simulink model "Copy_of_modelo_completo_sin_joystick"  (R2021a)
settings: Solver=FixedStepAuto  StartTime=0.0  StopTime=inf  FixedStep=0.001  MaxStep=1e-4  RelTol=1e-3
undefined symbols (not defined in the file): bah, bat, bcx, bcy, beqhd, beqt, bw, C_HEIGHT, cols_centers, cols_height, cont_mass, ddxmax, ddxmin, ddymax, ddymin, g, Kcy, Ksah, Ksat, Ksiah, Ksiat, Kw, lh0, Meqh, Meqt, mt, Rd, rt, rth, Rw, sigbuilder_block, sp_mass, VH_MAX, VT_MAX, w_mt_h, w_mt_i, xmax, xt0, ymax, yt0
libraries: simulink x1
(part 1 of 2)
settings Model: Creator=Mariano  LastModifiedBy=Mariano
settings SolverCC: ODENIntegrationMethod=ode2

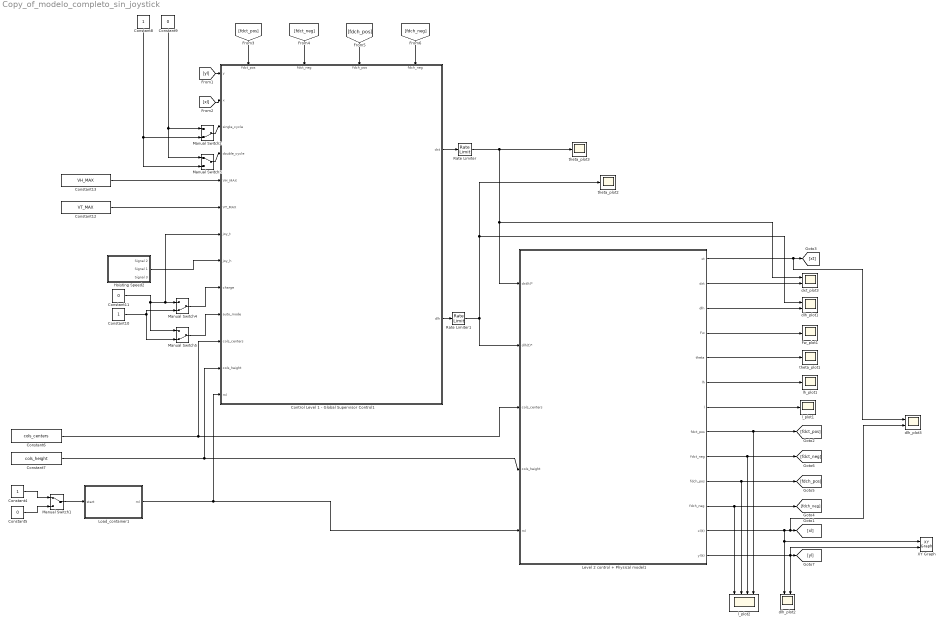
== system Copy_of_modelo_completo_sin_joystick ==
  Constant10 : Constant
  Constant11 : Constant  Value=0
  Constant12 : Constant  Value=VT_MAX
  Constant13 : Constant  Value=VH_MAX
  Constant4 : Constant
  Constant5 : Constant  Value=0
  Constant6 : Constant  Value=cols_centers
  Constant7 : Constant  Value=cols_height
  Constant8 : Constant
  Constant9 : Constant  Value=0
  Control Level 1 - Global Supervisor Control1 : Stateflow chart  TreatAsAtomicUnit=on
      settings: PortSchema="{\"entries\":[{\"content\":{\"sides\":[{\"content\":{\"connectorIds\":[\"In5\",\"In9\",\"In10\",\"In11\",\"In12\",\"In13\",\"In6\",\"In7\",\"In14\",\"In8\",\"In15\",\"In16\",\"In17\"]},\"type\":\"ConnectorPlacement.EquallySpacedRectSide\",\"uuid\":\"6e151bdd-c3d8-41a7-9f18-e2357f64189a\"},{\"content\":{\"connectorIds\":[\"Out1\",\"Out2\"],\"side\":\"RIGHT\"},\"type\":\"ConnectorPlacement.EquallySpacedRectSide\",\"uuid\":\"a3c41cfb-ae11-4b18-951d-06971f73a30a\"},{\"content\":{\"connectorIds\":[\"In1\",\"In2\",\"In3\",\"In4\"],\"side\":\"TOP\"},\"type\":\"ConnectorPlacement.EquallySpacedRectSide\",\"uuid\":\"cee4e257-0e1b-4274-aa91-a6c4290c0560\"},{\"content\":{\"connectorIds\":[],\"side\":\"BOTTOM\"},\"type\":\"ConnectorPlacement.EquallySpacedRectSide\",\"uuid\":\"f9084d8a-5b88-4444-9be3-56009c74d696\"}]},\"type\":\"ConnectorPlacement.EquallySpacedConnector\",\"uuid\":\"a9a1dd87-5328-46c3-9f4f-ca95d008ff72\"}],\"packageUris\":[\"http://schema.mathworks.com/mf0/Connector/R2020b\"],\"version\":\"1.0\"}"
  Fw_plot1 : Scope
  Hoisting Speed2 : Subsystem  Tag=STV Subsys  LoadFcn=sigbuilder_block('load',[0 30 1024.5 488.25 ]);  StartFcn=sigbuilder_block('start');  StopFcn=sigbuilder_block('stop');  ClipboardFcn=sigbuilder_block('clipboard');  mask(Sigbuilder block){tuvar=[0:10]}
      mask help: Simulink:masks:SigbuilderBlock_MD
      mask init:
      | if ~strcmp(get_param(bdroot(gcbh),'SimulationStatus'),'stopped') tuvar = sigbuilder_block('maskInit'); end
      settings: CopyFcn=sigbuilder_block('copy');  DeleteFcn=sigbuilder_block('delete');  ModelCloseFcn=sigbuilder_block('modelClose');  PreSaveFcn=sigbuilder_block('preSave');  PauseFcn=sigbuilder_block('pause');  ContinueFcn=sigbuilder_block('continue');  NameChangeFcn=sigbuilder_block('namechange');  OpenFcn=sigbuilder_block('open',[6 30 1012.5 447.75 ]);  CloseFcn=sigbuilder_block('close');
      mask Display: plot(0, 0, 100, 100,[2, 2, 32, 32, 2], [68, 8, 8, 68, 68],[32, 2], [38, 38], [32, 19, 2],[53, 60, 44], [32, 17, 17, 2],[16, 16, 31, 31]);txt = getActiveGroup(gcbh);text(2, 100, txt,'verticalAlignment', 'top');
  Level 2 control + Physical model1 : Subsystem
  Load_container1 : Subsystem
  Manual Switch1 : ManualSwitch
  Manual Switch2 : ManualSwitch  CurrentSetting=0
  Manual Switch3 : ManualSwitch
  Manual Switch4 : ManualSwitch  CurrentSetting=0
  Manual Switch5 : ManualSwitch  CurrentSetting=0
  Rate Limiter : RateLimiter  RisingSlewLimit=ddxmax  FallingSlewLimit=ddxmin  SampleTimeMode=inherited
  Rate Limiter1 : RateLimiter  RisingSlewLimit=ddymax  FallingSlewLimit=ddymin  SampleTimeMode=inherited
  XY Graph : simulink/Sinks/XY Graph  xmin=-20  xmax=60  ymin=-20  ymax=50  st=-1
  dlh_plot1 : Scope  NumInputPorts=2
  dlh_plot2 : Scope  NumInputPorts=2
  dlh_plot3 : Scope  NumInputPorts=2
  dxt_plot3 : Scope  NumInputPorts=2
  l_plot1 : Scope
  l_plot2 : Scope  NumInputPorts=4
  lh_plot1 : Scope
  theta_plot1 : Scope
  theta_plot2 : Scope
  theta_plot3 : Scope
  wires:
  [yl] -> Control Level 1 - Global Supervisor Control1/5(y)
  Manual Switch4/1 -> Control Level 1 - Global Supervisor Control1/14(charge)
  Constant11/1 -> Manual Switch5/1, Control Level 1 - Global Supervisor Control1/6(joy_t), Manual Switch4/1
  Constant9/1 -> Manual Switch3/1, Manual Switch2/1
  Manual Switch3/1 -> Control Level 1 - Global Supervisor Control1/11(double_cycle)
  Constant8/1 -> Manual Switch3/2, Manual Switch2/2
  Constant7/1 -> Level 2 control + Physical model1/4(cols_height), Control Level 1 - Global Supervisor Control1/16(cols_height)
  Constant10/1 -> Manual Switch4/2, Manual Switch5/2
  Manual Switch2/1 -> Control Level 1 - Global Supervisor Control1/10(single_cycle)
  Level 2 control + Physical model1/5(theta) -> theta_plot1/1
  Manual Switch5/1 -> Control Level 1 - Global Supervisor Control1/8(auto_mode)
  Constant5/1 -> Manual Switch1/2
  Constant13/1 -> Control Level 1 - Global Supervisor Control1/12(VH_MAX)
  Level 2 control + Physical model1/7(l) -> l_plot1/1
  Level 2 control + Physical model1/2(dxt) -> dxt_plot3/2
  Level 2 control + Physical model1/1(xt) -> dlh_plot3/1, [xt]
  Level 2 control + Physical model1/4(Fw) -> Fw_plot1/1
  Load_container1/1(ml) -> Control Level 1 - Global Supervisor Control1/17(ml), Level 2 control + Physical model1/5(ml)
  Constant12/1 -> Control Level 1 - Global Supervisor Control1/13(VT_MAX)
  Constant4/1 -> Manual Switch1/1
  Manual Switch1/1 -> Load_container1/1(start)
  [xl] -> Control Level 1 - Global Supervisor Control1/9(x)
  Level 2 control + Physical model1/3(dlh) -> dlh_plot1/2
  Level 2 control + Physical model1/6(lh) -> lh_plot1/1
  Constant6/1 -> Level 2 control + Physical model1/3(cols_centers), Control Level 1 - Global Supervisor Control1/15(cols_centers)
  Control Level 1 - Global Supervisor Control1/2(dlh) -> Rate Limiter1/1
  Control Level 1 - Global Supervisor Control1/1(dxt) -> Rate Limiter/1
  Level 2 control + Physical model1/8(fdct_pos) -> l_plot2/4, [fdct_pos]
  Level 2 control + Physical model1/9(fdct_neg) -> l_plot2/3, [fdct_neg]
  Level 2 control + Physical model1/10(fdch_pos) -> l_plot2/2, [fdch_pos]
  Level 2 control + Physical model1/11(fdch_neg) -> l_plot2/1, [fdch_neg]
  [fdct_pos] -> Control Level 1 - Global Supervisor Control1/1(fdct_pos)
  [fdct_neg] -> Control Level 1 - Global Supervisor Control1/2(fdct_neg)
  [fdch_pos] -> Control Level 1 - Global Supervisor Control1/3(fdch_pos)
  [fdch_neg] -> Control Level 1 - Global Supervisor Control1/4(fdch_neg)
  Level 2 control + Physical model1/13(yl(t)) -> XY Graph/2, dlh_plot2/2, [yl]
  Level 2 control + Physical model1/12(xl(t)) -> dlh_plot3/2, [xl], XY Graph/1, dlh_plot2/1
  Rate Limiter/1 -> theta_plot3/1, dxt_plot3/1, Level 2 control + Physical model1/1(dxt(t)*)
  Rate Limiter1/1 -> Level 2 control + Physical model1/2(dlh(t)*), theta_plot2/1, dlh_plot1/1
  Hoisting Speed2/2(Signal 1) -> Control Level 1 - Global Supervisor Control1/7(joy_h)

== system Copy_of_modelo_completo_sin_joystick/Hoisting Speed2 ==
  Demux : Demux  Tag=STV Demux  Outputs=3
      settings: DisplayOption=none
  FromWs : FromWorkspace  Tag=STV FromWs  VariableName=tuvar
      SigBuilderData=|
      | common.afterFinalStr = 'Extrapolate'
      | common.sampleTime = 0
      | dataSet.timeRange = [0 105]
      | dataSet.name = 'Group 1'
      | sbobj.Groups.Name = 'Group 1'
      | sbobj.Groups.Signals(1).Name = 'Signal 2'
      | sbobj.Groups.Signals(1).XData = [0 5 8 52 55 105]
      | sbobj.Groups.Signals(1).YData = [0 0 -1 -1 0 0]
      | sbobj.Groups.Signals(2).Name = 'Signal 1'
      | sbobj.Groups.Signals(2).XData = [0 2 4 20 22 34 36 48 50 105]
      | sbobj.Groups.Signals(2).YData = [0 0 -1 -1 0 0 1 1 0 0]
      | sbobj.Groups.Signals(3).Name = 'Signal 3'
      | sbobj.Groups.Signals(3).XData = [0 8 10 30.1 32 105]
      | sbobj.Groups.Signals(3).YData = [0 0 1 1 0 0]
      | sbobj.Groups.TimeRange = [0 105]
  Signal 2 : Outport  Tag=STV Outport
  Signal 1 : Outport  Tag=STV Outport  Port=2
  Signal 3 : Outport  Tag=STV Outport  Port=3
  wires:
  FromWs/1 -> Demux/1
  Demux/1 -> Signal 2/1
  Demux/2 -> Signal 1/1
  Demux/3 -> Signal 3/1

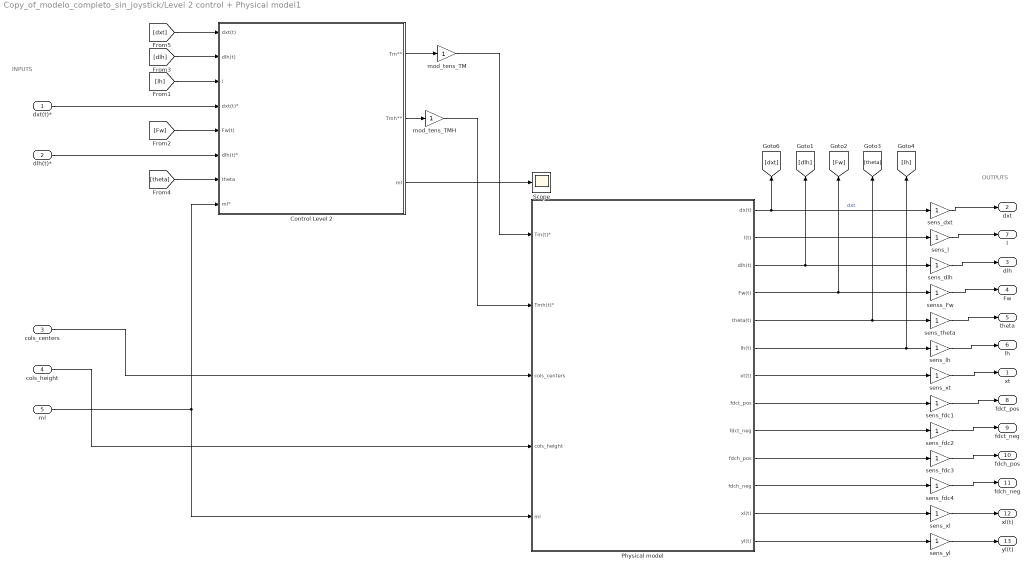
== system Copy_of_modelo_completo_sin_joystick/Level 2 control + Physical model1 ==
  note: OUTPUTS
  note: INPUTS
  dxt(t)* : Inport
  dlh(t)* : Inport  Port=2
  cols_centers : Inport  Port=3
  cols_height : Inport  Port=4
  ml : Inport  Port=5
  Control Level 2 : Subsystem
  Physical model : Subsystem
  Scope : Scope
  mod_tens_TM : Gain
  mod_tens_TMH : Gain
  sens_dlh : Gain
  sens_dxt : Gain
  sens_fdc{1..4} (4 alike) : Gain
  sens_l : Gain
  sens_lh : Gain
  sens_theta : Gain
  sens_xl : Gain
  sens_xt : Gain
  sens_yl : Gain
  senss_Fw : Gain
  xt : Outport
  dxt : Outport  Port=2
  dlh : Outport  Port=3
  Fw : Outport  Port=4
  theta : Outport  Port=5
  lh : Outport  Port=6
  l : Outport  Port=7
  fdct_pos : Outport  Port=8
  fdct_neg : Outport  Port=9
  fdch_pos : Outport  Port=10
  fdch_neg : Outport  Port=11
  xl(t) : Outport  Port=12
  yl(t) : Outport  Port=13
  wires:
  Physical model/4(Fw(t)) -> senss_Fw/1, [Fw]
  Physical model/3(dlh(t)) -> sens_dlh/1, [dlh]
  dxt(t)*/1 -> Control Level 2/4(dxt(t)*)
  senss_Fw/1 -> Fw/1
  Control Level 2/3(ml) -> Scope/1
  sens_xt/1 -> xt/1
  dlh(t)*/1 -> Control Level 2/6(dlh(t)*)
  Physical model/5(theta(t)) -> sens_theta/1, [theta]
  mod_tens_TMH/1 -> Physical model/2(Tmh(t)*)
  Physical model/1(dx(t)) -> sens_dxt/1, [dxt]  "dxt"
  ml/1 -> Physical model/5(ml), Control Level 2/8(ml*)
  Physical model/6(lh(t)) -> sens_lh/1, [lh]
  sens_dlh/1 -> dlh/1
  sens_theta/1 -> theta/1
  Control Level 2/1(Tm**) -> mod_tens_TM/1
  Physical model/2(l(t)) -> sens_l/1
  sens_lh/1 -> lh/1
  sens_dxt/1 -> dxt/1
  Physical model/7(xt(t)) -> sens_xt/1
  Control Level 2/2(Tmh**) -> mod_tens_TMH/1
  mod_tens_TM/1 -> Physical model/1(Tm(t)*)
  cols_centers/1 -> Physical model/3(cols_centers)
  cols_height/1 -> Physical model/4(cols_height)
  sens_l/1 -> l/1
  [dxt] -> Control Level 2/1(dxt(t))
  [lh] -> Control Level 2/3(l)
  [Fw] -> Control Level 2/5(Fw(t))
  [dlh] -> Control Level 2/2(dlh(t))
  [theta] -> Control Level 2/7(theta)
  sens_fdc1/1 -> fdct_pos/1
  Physical model/8(fdct_pos) -> sens_fdc1/1
  sens_fdc4/1 -> fdch_neg/1
  sens_fdc3/1 -> fdch_pos/1
  sens_fdc2/1 -> fdct_neg/1
  Physical model/9(fdct_neg) -> sens_fdc2/1
  Physical model/10(fdch_pos) -> sens_fdc3/1
  Physical model/11(fdch_neg) -> sens_fdc4/1
  Physical model/13(yl(t)) -> sens_yl/1
  Physical model/12(xl(t)) -> sens_xl/1
  sens_xl/1 -> xl(t)/1
  sens_yl/1 -> yl(t)/1

== system Copy_of_modelo_completo_sin_joystick/Load_container1 ==
  start : Inport
  Sum : Sum  Inputs=|++
  Switch : Switch  Criteria=u2 > Threshold
  no_container : Constant  Value=cont_mass
  random_container_mass : Constant  Value=cont_mass
  spreader mass : Constant  Value=sp_mass
  ml : Outport
  wires:
  no_container/1 -> Switch/1
  spreader mass/1 -> Sum/2
  random_container_mass/1 -> Switch/3
  Switch/1 -> Sum/1
  Sum/1 -> ml/1
  start/1 -> Switch/2

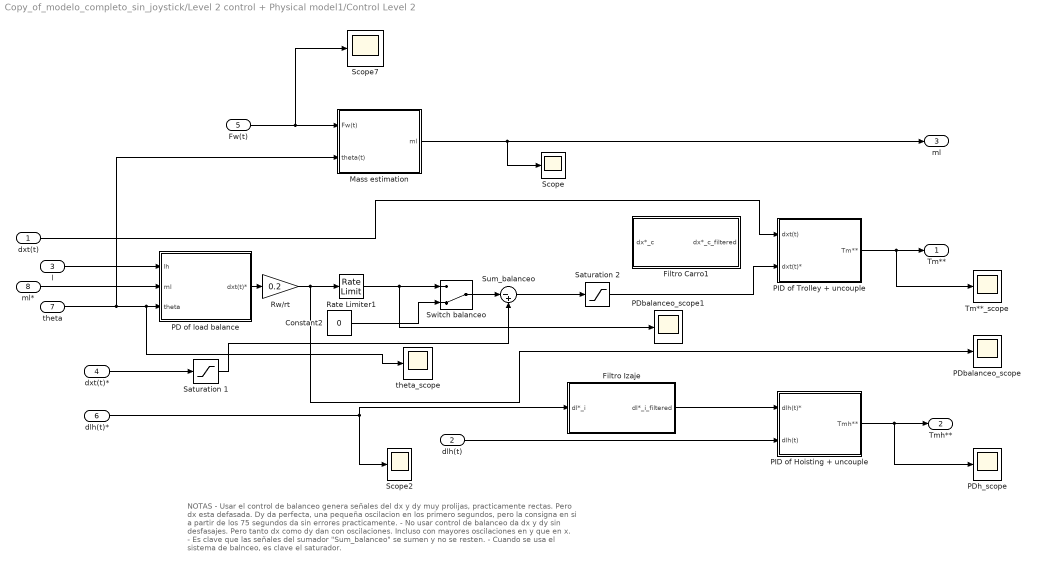
== system Copy_of_modelo_completo_sin_joystick/Level 2 control + Physical model1/Control Level 2 ==
  note: NOTAS
      | - Usar el control de balanceo genera señales del dx y dy muy prolijas, practicamente rectas. Pero dx esta
      | defasada. Dy da perfecta, una pequeña oscilacion en los primero segundos, pero la consigna en si a partir
      | de los 75 segundos da sin errores practicamente.
      |
      | - No usar control de balanceo da dx y dy sin desfasajes. Pero tanto dx como dy dan con oscilaciones. Incluso
      | con mayores oscilaciones en y que en x.
      |
      | - Es clave que las señales del sumador "Sum_balanceo" se sumen y no se resten.
      |
      | - Cuando se usa el sistema de balnceo, es clave el saturador.
  dxt(t) : Inport
  dlh(t) : Inport  Port=2
  l : Inport  Port=3
  dxt(t)* : Inport  Port=4
  Fw(t) : Inport  Port=5
  dlh(t)* : Inport  Port=6
  theta : Inport  Port=7
  ml* : Inport  Port=8
  Constant2 : Constant  Value=0
  Filtro Carro1 : Subsystem
  Filtro Izaje : Subsystem
  Mass estimation : Subsystem
  "PD of load balance " : Subsystem
  PDbalanceo_scope : Scope
  PDbalanceo_scope1 : Scope
  PDh_scope : Scope
  "PID of Hoisting + uncouple " : Subsystem
  "PID of Trolley + uncouple " : Subsystem
  Rate Limiter1 : RateLimiter  RisingSlewLimit=ddymax  FallingSlewLimit=ddymin  SampleTimeMode=inherited
  Rw/rt : Gain  Gain=0.2
  Saturation 1 : Saturate  UpperLimit=4  LowerLimit=-4  ZeroCross=off
  Saturation 2 : Saturate  UpperLimit=4  LowerLimit=-4  ZeroCross=off
  Scope : Scope
  Scope2 : Scope
  Scope7 : Scope
  Sum_balanceo : Sum  Inputs=|-+
  Switch balanceo : ManualSwitch  CurrentSetting=0
  Tm**_scope : Scope
  theta_scope : Scope
  Tm** : Outport
  Tmh** : Outport  Port=2
  ml : Outport  Port=3
  wires:
  Fw(t)/1 -> Scope7/1, Mass estimation/1(Fw(t))
  "PID of Trolley + uncouple "/1(Tm**) -> Tm**_scope/1, Tm**/1
  Mass estimation/1(ml) -> Scope/1, ml/1
  dxt(t)/1 -> "PID of Trolley + uncouple "/1(dxt(t))
  "PID of Hoisting + uncouple "/1(Tmh**) -> PDh_scope/1, Tmh**/1
  l/1 -> "PD of load balance "/1(lh)
  theta/1 -> Mass estimation/2(theta(t)), "PD of load balance "/3(theta), theta_scope/1
  dlh(t)/1 -> "PID of Hoisting + uncouple "/2(dlh(t))
  dlh(t)*/1 -> Filtro Izaje/1(dl*_i), Scope2/1
  "PD of load balance "/1(dxt(t)*) -> Rw/rt/1
  ml*/1 -> "PD of load balance "/2(ml)
  Constant2/1 -> Switch balanceo/2
  Filtro Izaje/1(dl*_i_filtered) -> "PID of Hoisting + uncouple "/1(dlh(t)*)
  Sum_balanceo/1 -> Saturation 2/1
  Switch balanceo/1 -> Sum_balanceo/1
  dxt(t)*/1 -> Saturation 1/1
  Saturation 1/1 -> Sum_balanceo/2
  Rw/rt/1 -> Rate Limiter1/1, PDbalanceo_scope/1
  Saturation 2/1 -> "PID of Trolley + uncouple "/2(dxt(t)*)
  Rate Limiter1/1 -> PDbalanceo_scope1/1, Switch balanceo/1

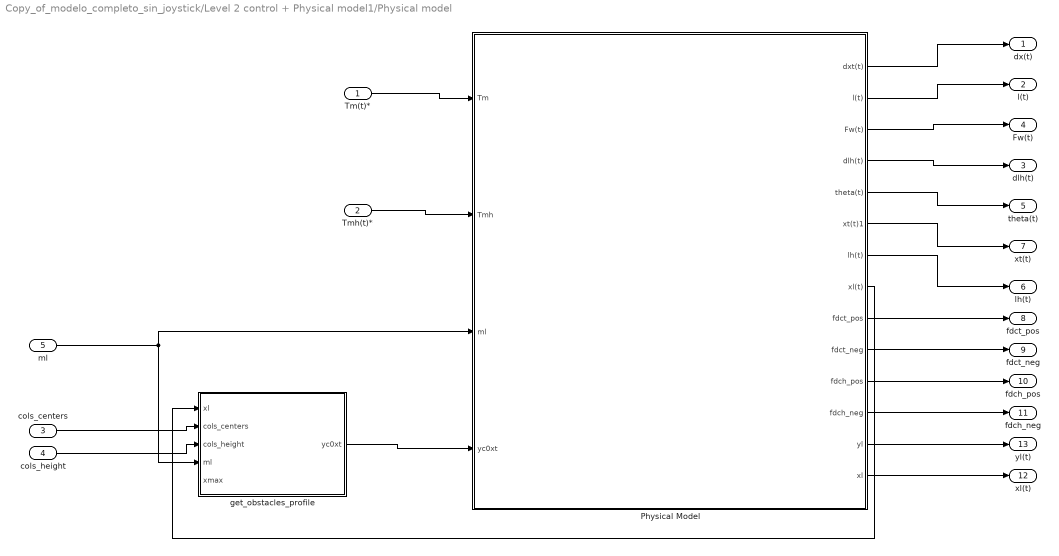
== system Copy_of_modelo_completo_sin_joystick/Level 2 control + Physical model1/Physical model ==
  Tm(t)* : Inport
  Tmh(t)* : Inport  Port=2
  cols_centers : Inport  Port=3
  cols_height : Inport  Port=4
  ml : Inport  Port=5
  Physical Model : Subsystem
  get_obstacles_profile : MATLAB Function  TreatAsAtomicUnit=on
  dx(t) : Outport
  l(t) : Outport  Port=2
  dlh(t) : Outport  Port=3
  Fw(t) : Outport  Port=4
  theta(t) : Outport  Port=5
  lh(t) : Outport  Port=6
  xt(t) : Outport  Port=7
  fdct_pos : Outport  Port=8
  fdct_neg : Outport  Port=9
  fdch_pos : Outport  Port=10
  fdch_neg : Outport  Port=11
  xl(t) : Outport  Port=12
  yl(t) : Outport  Port=13
  wires:
  Physical Model/4(dlh(t)) -> dlh(t)/1
  Physical Model/2(l(t)) -> l(t)/1
  Physical Model/1(dxt(t)) -> dx(t)/1
  Physical Model/3(Fw(t)) -> Fw(t)/1
  Physical Model/5(theta(t)) -> theta(t)/1
  Physical Model/6(xt(t)1) -> xt(t)/1
  Physical Model/7(lh(t)) -> lh(t)/1
  Tmh(t)*/1 -> Physical Model/2(Tmh)
  Tm(t)*/1 -> Physical Model/1(Tm)
  ml/1 -> get_obstacles_profile/4(ml), Physical Model/3(ml)
  get_obstacles_profile/1(yc0xt) -> Physical Model/4(yc0xt)
  Physical Model/8(xl(t)) -> get_obstacles_profile/1(xl)
  cols_centers/1 -> get_obstacles_profile/2(cols_centers)
  cols_height/1 -> get_obstacles_profile/3(cols_height)
  Physical Model/9(fdct_pos) -> fdct_pos/1
  Physical Model/10(fdct_neg) -> fdct_neg/1
  Physical Model/11(fdch_pos) -> fdch_pos/1
  Physical Model/12(fdch_neg) -> fdch_neg/1
  Physical Model/14(xl) -> xl(t)/1
  Physical Model/13(yl) -> yl(t)/1

== system Copy_of_modelo_completo_sin_joystick/Level 2 control + Physical model1/Control Level 2/Filtro Carro1 ==
  dx*_c : Inport
  2 : Gain  Gain=5
  Rate Limiter1 : RateLimiter  RisingSlewLimit=ddymax  FallingSlewLimit=ddymin  SampleTimeMode=inherited
  Sum3 : Sum  Inputs=|+-
  dl_h(t)2 : Integrator
  dx*_c_filtered : Outport  VectorParamsAs1DForOutWhenUnconnected=off
  wires:
  Sum3/1 -> dl_h(t)2/1
  2/1 -> dx*_c_filtered/1, Sum3/2
  dx*_c/1 -> Rate Limiter1/1
  dl_h(t)2/1 -> 2/1
  Rate Limiter1/1 -> Sum3/1

== system Copy_of_modelo_completo_sin_joystick/Level 2 control + Physical model1/Control Level 2/Filtro Izaje ==
  dl*_i : Inport
  1 : Gain  Gain=10
  Rate Limiter1 : RateLimiter  RisingSlewLimit=ddymax  FallingSlewLimit=ddymin  SampleTimeMode=inherited
  Sum4 : Sum  Inputs=|+-
  dl_h(t)1 : Integrator
  dl*_i_filtered : Outport  VectorParamsAs1DForOutWhenUnconnected=off
  wires:
  dl_h(t)1/1 -> 1/1
  1/1 -> dl*_i_filtered/1, Sum4/2
  Sum4/1 -> dl_h(t)1/1
  dl*_i/1 -> Rate Limiter1/1
  Rate Limiter1/1 -> Sum4/1

== system Copy_of_modelo_completo_sin_joystick/Level 2 control + Physical model1/Control Level 2/Mass estimation ==
  Fw(t) : Inport
  theta(t) : Inport  Port=2
  Constant : Constant  Value=g
  Divide : Product  Inputs=*/
  Product : Product
  Trigonometric Function : Trigonometry
  ml : Outport
  wires:
  theta(t)/1 -> Trigonometric Function/1
  Trigonometric Function/1 -> Product/2
  Fw(t)/1 -> Product/1
  Divide/1 -> ml/1
  Product/1 -> Divide/1
  Constant/1 -> Divide/2

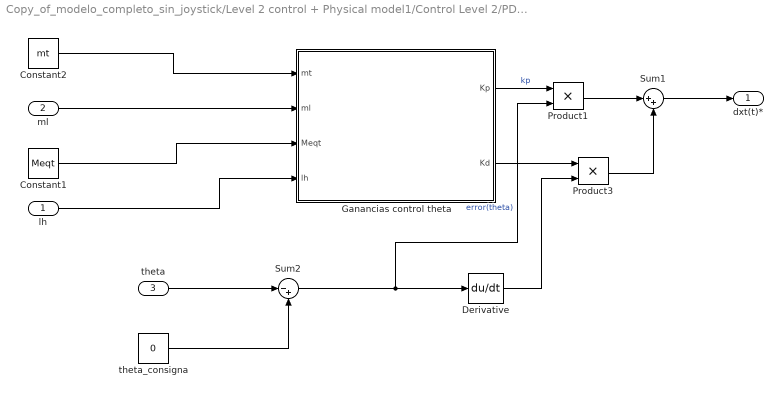
== system Copy_of_modelo_completo_sin_joystick/Level 2 control + Physical model1/Control Level 2/PD of load balance  ==
  lh : Inport
  ml : Inport  Port=2
  theta : Inport  Port=3
  Constant1 : Constant  Value=Meqt
  Constant2 : Constant  Value=mt
  Derivative : Derivative
  Ganancias control theta : MATLAB Function  TreatAsAtomicUnit=on
  Product1 : Product
  Product3 : Product
  Sum1 : Sum  Inputs=|++
  Sum2 : Sum  Inputs=|-+
  theta_consigna : Constant  Value=0
  dxt(t)* : Outport
  wires:
  ml/1 -> Ganancias control theta/2(ml)
  lh/1 -> Ganancias control theta/4(lh)
  Sum1/1 -> dxt(t)*/1
  Constant2/1 -> Ganancias control theta/1(mt)
  Constant1/1 -> Ganancias control theta/3(Meqt)
  Ganancias control theta/2(Kd) -> Product3/1
  Derivative/1 -> Product3/2
  Product3/1 -> Sum1/2
  Sum2/1 -> Derivative/1, Product1/2  "error(theta)"
  Product1/1 -> Sum1/1
  Ganancias control theta/1(Kp) -> Product1/1  "kp"
  theta/1 -> Sum2/1
  theta_consigna/1 -> Sum2/2

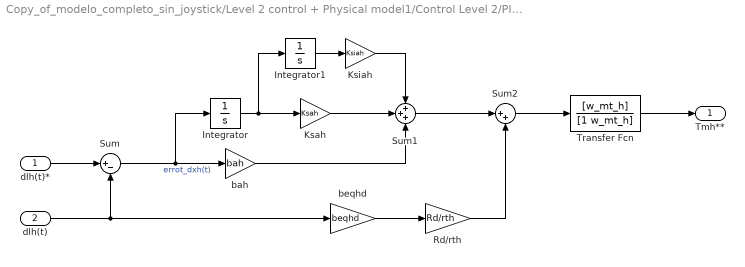
== system Copy_of_modelo_completo_sin_joystick/Level 2 control + Physical model1/Control Level 2/PID of Hoisting + uncouple  ==
  dlh(t)* : Inport
  dlh(t) : Inport  Port=2
  Integrator : Integrator
  Integrator1 : Integrator
  Ksah : Gain  Gain=Ksah
  Ksiah : Gain  Gain=Ksiah
  Rd/rth : Gain  Gain=Rd/rth
  Sum : Sum  Inputs=|+-
  Sum1 : Sum  Inputs=+++
  Sum2 : Sum  Inputs=|++
  Transfer Fcn : TransferFcn  Numerator=[w_mt_h]  Denominator=[1 w_mt_h]
  bah : Gain  Gain=bah
  beqhd : Gain  Gain=beqhd
  Tmh** : Outport
  wires:
  Sum/1 -> bah/1, Integrator/1  "errot_dxh(t)"
  dlh(t)*/1 -> Sum/1
  Sum1/1 -> Sum2/1
  dlh(t)/1 -> Sum/2, beqhd/1
  Integrator/1 -> Integrator1/1, Ksah/1
  bah/1 -> Sum1/3
  Ksah/1 -> Sum1/2
  Integrator1/1 -> Ksiah/1
  Ksiah/1 -> Sum1/1
  beqhd/1 -> Rd/rth/1
  Sum2/1 -> Transfer Fcn/1
  Rd/rth/1 -> Sum2/2
  Transfer Fcn/1 -> Tmh**/1

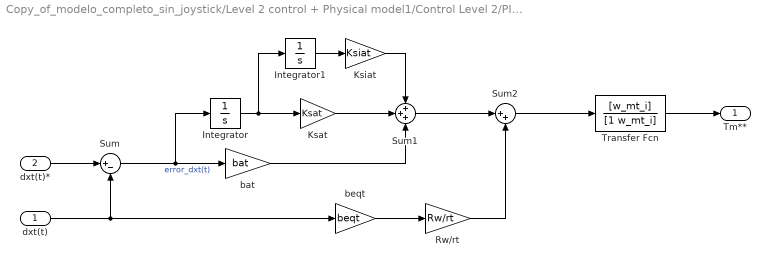
== system Copy_of_modelo_completo_sin_joystick/Level 2 control + Physical model1/Control Level 2/PID of Trolley + uncouple  ==
  dxt(t) : Inport
  dxt(t)* : Inport  Port=2
  Integrator : Integrator
  Integrator1 : Integrator
  Ksat : Gain  Gain=Ksat
  Ksiat : Gain  Gain=Ksiat
  Rw/rt : Gain  Gain=Rw/rt
  Sum : Sum  Inputs=|+-
  Sum1 : Sum  Inputs=+++
  Sum2 : Sum  Inputs=|++
  Transfer Fcn : TransferFcn  Numerator=[w_mt_i]  Denominator=[1 w_mt_i]
  bat : Gain  Gain=bat
  beqt : Gain  Gain=beqt
  Tm** : Outport
  wires:
  Sum/1 -> bat/1, Integrator/1  "error_dxt(t)"
  dxt(t)*/1 -> Sum/1
  dxt(t)/1 -> Sum/2, beqt/1
  Integrator/1 -> Integrator1/1, Ksat/1
  bat/1 -> Sum1/3
  Ksat/1 -> Sum1/2
  Integrator1/1 -> Ksiat/1
  Ksiat/1 -> Sum1/1
  beqt/1 -> Rw/rt/1
  Sum1/1 -> Sum2/1
  Rw/rt/1 -> Sum2/2
  Sum2/1 -> Transfer Fcn/1
  Transfer Fcn/1 -> Tm**/1

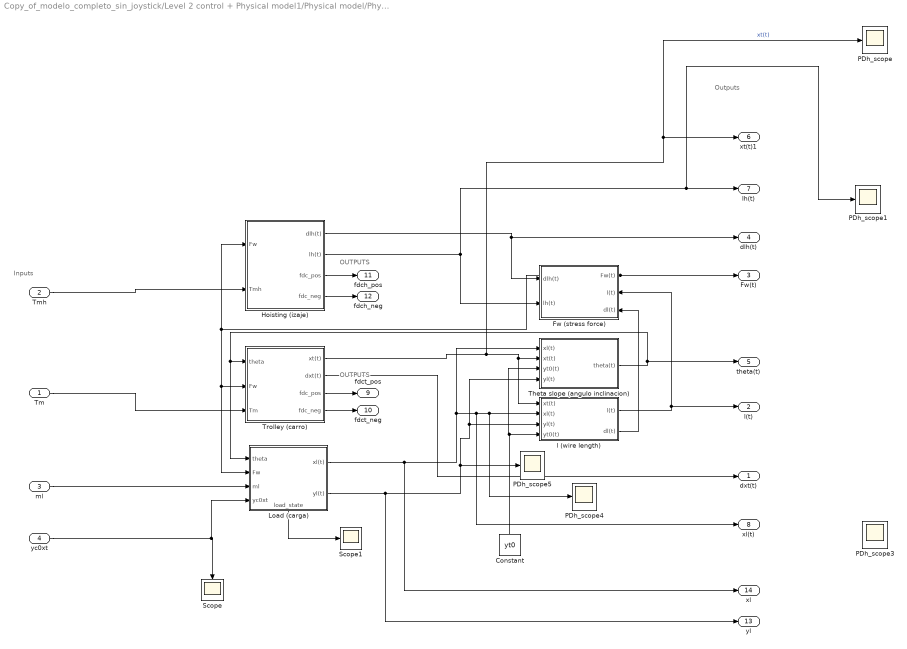
== system Copy_of_modelo_completo_sin_joystick/Level 2 control + Physical model1/Physical model/Physical Model ==
  note: OUTPUTS
  note: Inputs
  note: Outputs
  note: OUTPUTS
  Tm : Inport
  Tmh : Inport  Port=2
  ml : Inport  Port=3
  yc0xt : Inport  Port=4
  Constant : Constant  Value=yt0
  Fw (stress force) : Subsystem
      settings: PortSchema="{\"entries\":[{\"content\":{\"sides\":[{\"content\":{\"connectorIds\":[\"In1\",\"In2\"]},\"type\":\"ConnectorPlacement.EquallySpacedRectSide\",\"uuid\":\"ba23d8a5-df88-4a98-9228-1a95ef0572d6\"},{\"content\":{\"connectorIds\":[\"Out1\",\"In3\",\"In4\"],\"side\":\"RIGHT\"},\"type\":\"ConnectorPlacement.EquallySpacedRectSide\",\"uuid\":\"c1b2cc2a-1d19-40da-89ec-405abbf25b58\"},{\"content\":{\"connectorIds\":[],\"side\":\"TOP\"},\"type\":\"ConnectorPlacement.EquallySpacedRectSide\",\"uuid\":\"8c283652-7118-429a-8320-3bc0966db205\"}]},\"type\":\"ConnectorPlacement.EquallySpacedConnector\",\"uuid\":\"7ebc4a5f-6f80-4333-9ee6-9a21b2f2a5d0\"}],\"packageUris\":[\"http://schema.mathworks.com/mf0/Connector/R2020b\"],\"version\":\"1.0\"}"
  Hoisting (izaje) : Subsystem
  Load (carga) : Subsystem
      settings: PortSchema="{\"entries\":[{\"content\":{\"sides\":[{\"content\":{\"connectorIds\":[\"In1\",\"In2\",\"In3\",\"In4\"]},\"type\":\"ConnectorPlacement.EquallySpacedRectSide\",\"uuid\":\"37592506-3a6b-4567-92e8-42290e8eeea3\"},{\"content\":{\"connectorIds\":[\"Out1\",\"Out2\"],\"side\":\"RIGHT\"},\"type\":\"ConnectorPlacement.EquallySpacedRectSide\",\"uuid\":\"0ecb02fc-3423-4f4d-ad91-2cd2f59fe210\"},{\"content\":{\"connectorIds\":[],\"side\":\"TOP\"},\"type\":\"ConnectorPlacement.EquallySpacedRectSide\",\"uuid\":\"e98f0cef-87c8-4aed-91c0-03b7690ae30e\"},{\"content\":{\"connectorIds\":[\"Out3\"],\"side\":\"BOTTOM\"},\"type\":\"ConnectorPlacement.EquallySpacedRectSide\",\"uuid\":\"e16fbcf8-4df1-4bb9-aaa8-254f3178aeca\"}]},\"type\":\"ConnectorPlacement.EquallySpacedConnector\",\"uuid\":\"38642e74-d943-4236-849b-c2d295c3b31e\"}],\"packageUris\":[\"http://schema.mathworks.com/mf0/Connector/R2020b\"],\"version\":\"1.0\"}"
  PDh_scope{,1,3..5} (5 alike) : Scope
  Scope : Scope
  Scope1 : Scope
  Theta slope (angulo inclinacion) : Subsystem
  Trolley (carro) : Subsystem
  l (wire length) : Subsystem
  dxt(t) : Outport
  l(t) : Outport  Port=2
  Fw(t) : Outport  Port=3
  dlh(t) : Outport  Port=4
  theta(t) : Outport  Port=5
  xt(t)1 : Outport  Port=6
  lh(t) : Outport  Port=7
  xl(t) : Outport  Port=8
  fdct_pos : Outport  Port=9
  fdct_neg : Outport  Port=10
  fdch_pos : Outport  Port=11
  fdch_neg : Outport  Port=12
  yl : Outport  Port=13
  xl : Outport  Port=14
  wires:
  Theta slope (angulo inclinacion)/1(theta(t)) -> theta(t)/1, Load (carga)/1(theta), Trolley (carro)/1(theta)
  Load (carga)/1(xl(t)) -> xl/1, xl(t)/1, PDh_scope4/1, l (wire length)/2(xl(t)), Theta slope (angulo inclinacion)/1(xl(t))
  Hoisting (izaje)/2(lh(t)) -> Fw (stress force)/2(lh(t)), PDh_scope1/1, lh(t)/1
  Trolley (carro)/1(xt(t)) -> PDh_scope/1, xt(t)1/1, l (wire length)/1(xt(t)), Theta slope (angulo inclinacion)/2(xt(t))  "xt(t)"
  Fw (stress force)/1(Fw(t)) -> Fw(t)/1, Load (carga)/2(Fw), Trolley (carro)/2(Fw), Hoisting (izaje)/1(Fw)
  Constant/1 -> Theta slope (angulo inclinacion)/3(yt0(t)), l (wire length)/4(yt0(t))
  Load (carga)/2(yl(t)) -> yl/1, Theta slope (angulo inclinacion)/4(yl(t)), l (wire length)/3(yl(t)), PDh_scope5/1
  l (wire length)/1(l(t)) -> l(t)/1, Fw (stress force)/3(l(t))
  ml/1 -> Load (carga)/3(ml)
  l (wire length)/2(dl(t)) -> Fw (stress force)/4(dl(t))
  Tmh/1 -> Hoisting (izaje)/2(Tmh)
  Tm/1 -> Trolley (carro)/3(Tm)
  Hoisting (izaje)/1(dlh(t)) -> Fw (stress force)/1(dlh(t)), dlh(t)/1
  Trolley (carro)/2(dxt(t)) -> dxt(t)/1
  yc0xt/1 -> Load (carga)/4(yc0xt), Scope/1
  Load (carga)/3(load_state) -> Scope1/1
  Trolley (carro)/4(fdc_neg) -> fdct_neg/1
  Trolley (carro)/3(fdc_pos) -> fdct_pos/1
  Hoisting (izaje)/3(fdc_pos) -> fdch_pos/1
  Hoisting (izaje)/4(fdc_neg) -> fdch_neg/1

== system Copy_of_modelo_completo_sin_joystick/Level 2 control + Physical model1/Physical model/Physical Model/Fw (stress force) ==
  note: Carga suspendida
  note: Carga apoyada
  dlh(t) : Inport
  lh(t) : Inport  Port=2
  l(t) : Inport  Port=3
  dl(t) : Inport  Port=4
  Kw : Gain  Gain=Kw
  Kw2 : Gain  Gain=bw
  Sum1 : Sum  Inputs=|+-
  Sum2 : Sum  Inputs=|++
  Sum3 : Sum  Inputs=|+-
  Sum5 : Sum  Inputs=|+-
  Switch : Switch  Criteria=u2 > Threshold
  bw1 : Gain  Gain=bw
  Fw(t) : Outport
  wires:
  Switch/1 -> Fw(t)/1
  l(t)/1 -> Sum1/1
  lh(t)/1 -> Sum1/2
  Sum1/1 -> Switch/2, Kw/1
  Sum3/1 -> bw1/1
  bw1/1 -> Sum2/2
  Kw/1 -> Sum2/1
  Sum2/1 -> Switch/1
  Sum5/1 -> Kw2/1
  dlh(t)/1 -> Sum5/2, Sum3/2
  dl(t)/1 -> Sum5/1, Sum3/1
  Kw2/1 -> Switch/3

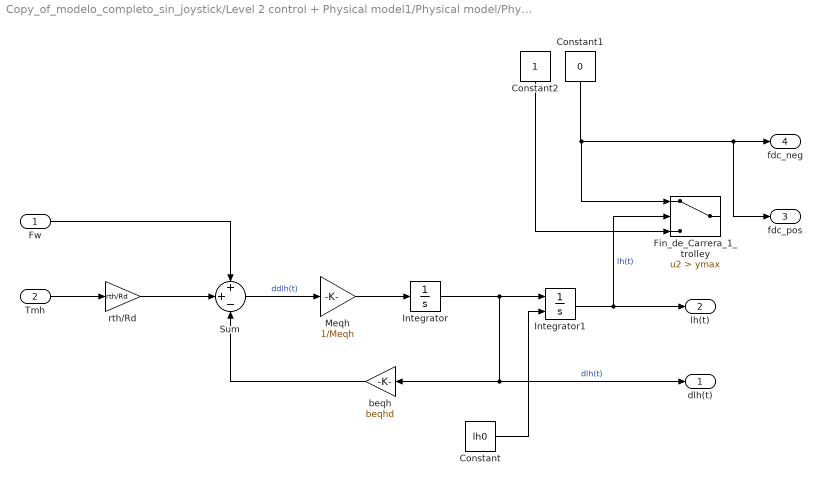
== system Copy_of_modelo_completo_sin_joystick/Level 2 control + Physical model1/Physical model/Physical Model/Hoisting (izaje) ==
  Fw : Inport
  Tmh : Inport  Port=2
  Constant : Constant  Value=lh0
  Constant1 : Constant  Value=0
  Constant2 : Constant
  Fin_de_Carrera_1_trolley : Switch  Criteria=u2 > Threshold  Threshold=ymax
  Integrator : Integrator
  Integrator1 : Integrator  InitialConditionSource=external
  Meqh : Gain  Gain=1/Meqh
  Sum : Sum  Inputs=++-
  beqh : Gain  Gain=beqhd
  rth/Rd : Gain  Gain=rth/Rd
  dlh(t) : Outport
  lh(t) : Outport  Port=2
  fdc_pos : Outport  Port=3
  fdc_neg : Outport  Port=4
  wires:
  Fw/1 -> Sum/1
  Tmh/1 -> rth/Rd/1
  rth/Rd/1 -> Sum/2
  Sum/1 -> Meqh/1  "ddlh(t)"
  Meqh/1 -> Integrator/1
  Integrator/1 -> dlh(t)/1, beqh/1, Integrator1/1  "dlh(t)"
  Integrator1/1 -> Fin_de_Carrera_1_trolley/2, lh(t)/1  "lh(t)"
  beqh/1 -> Sum/3
  Constant/1 -> Integrator1/2
  Constant1/1 -> Fin_de_Carrera_1_trolley/1, fdc_pos/1, fdc_neg/1
  Constant2/1 -> Fin_de_Carrera_1_trolley/3

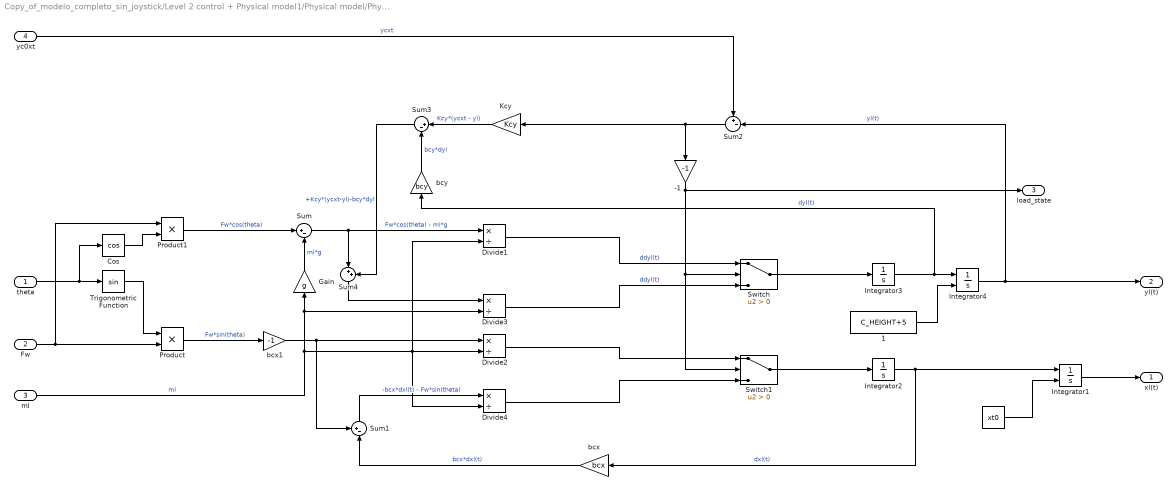
== system Copy_of_modelo_completo_sin_joystick/Level 2 control + Physical model1/Physical model/Physical Model/Load (carga) ==
  theta : Inport
  Fw : Inport  Port=2
  ml : Inport  Port=3
  yc0xt : Inport  Port=4
  "   " : Constant  Value=xt0
  "   1" : Constant  Value=C_HEIGHT+5
  -1 : Gain  Gain=-1
  Cos : Trigonometry  Operator=cos
  Divide{1..4} (4 alike) : Product  Inputs=*/
  Gain : Gain  Gain=g
  Integrator1 : Integrator  InitialConditionSource=external
  Integrator2 : Integrator
  Integrator3 : Integrator
  Integrator4 : Integrator  InitialConditionSource=external
  Kcy : Gain  Gain=Kcy
  Product : Product
  Product1 : Product
  Sum : Sum  Inputs=|+-
  Sum1 : Sum  Inputs=+-|
  Sum2 : Sum  Inputs=+-|
  Sum3 : Sum  Inputs=|+-
  Sum4 : Sum  Inputs=|++
  Switch : Switch  Criteria=u2 > Threshold
  Switch1 : Switch  Criteria=u2 > Threshold
  Trigonometric Function : Trigonometry
  bcx : Gain  Gain=bcx
  bcx1 : Gain  Gain=-1
  bcy : Gain  Gain=bcy
  xl(t) : Outport
  yl(t) : Outport  Port=2
  load_state : Outport  Port=3
  wires:
  theta/1 -> Trigonometric Function/1, Cos/1
  Trigonometric Function/1 -> Product/1
  Fw/1 -> Product/2, Product1/1
  Integrator1/1 -> xl(t)/1
  Integrator2/1 -> bcx/1, Integrator1/1  "dxl(t)"
  ml/1 -> Divide4/2, Divide2/2, Divide1/2, Divide3/2, Gain/1  "ml"
  Product/1 -> bcx1/1  "Fw*sin(theta)"
  Cos/1 -> Product1/2
  Product1/1 -> Sum/1  "Fw*cos(theta)"
  Sum/1 -> Sum4/1, Divide1/1  "Fw*cos(theta) - ml*g"
  Integrator3/1 -> bcy/1, Integrator4/1  "dyl(t)"
  Integrator4/1 -> Sum2/2, yl(t)/1  "yl(t)"
  Gain/1 -> Sum/2  "ml*g"
  Divide1/1 -> Switch/1  "ddyl(t)"
  Switch/1 -> Integrator3/1
  Switch1/1 -> Integrator2/1
  Divide2/1 -> Switch1/1
  Divide4/1 -> Switch1/3
  Divide3/1 -> Switch/3  "ddyl(t)"
  bcx1/1 -> Sum1/1, Divide2/1
  bcx/1 -> Sum1/2  "bcx*dxl(t)"
  Sum1/1 -> Divide4/1  "-bcx*dxl(t) - Fw*sin(theta)"
  Sum2/1 -> Kcy/1, -1/1
  yc0xt/1 -> Sum2/1  "ycxt"
  Kcy/1 -> Sum3/1  "Kcy*(ycxt - yl)"
  bcy/1 -> Sum3/2  "bcy*dyl"
  Sum4/1 -> Divide3/1
  Sum3/1 -> Sum4/2  "+Kcy*(ycxt-yl)-bcy*dyl"
  -1/1 -> load_state/1, Switch1/2, Switch/2
  "   "/1 -> Integrator1/2
  "   1"/1 -> Integrator4/2

== system Copy_of_modelo_completo_sin_joystick/Level 2 control + Physical model1/Physical model/Physical Model/Theta slope (angulo inclinacion) ==
  xl(t) : Inport
  xt(t) : Inport  Port=2
  yt0(t) : Inport  Port=3
  yl(t) : Inport  Port=4
  Atan2 : Trigonometry  Operator=atan2
  Sum : Sum  Inputs=+-
  Sum1 : Sum  Inputs=+-
  theta(t) : Outport
  wires:
  yt0(t)/1 -> Sum/1
  yl(t)/1 -> Sum/2
  xl(t)/1 -> Sum1/1
  xt(t)/1 -> Sum1/2
  Sum1/1 -> Atan2/1  "xl-xt"
  Sum/1 -> Atan2/2  "yl-yt"
  Atan2/1 -> theta(t)/1

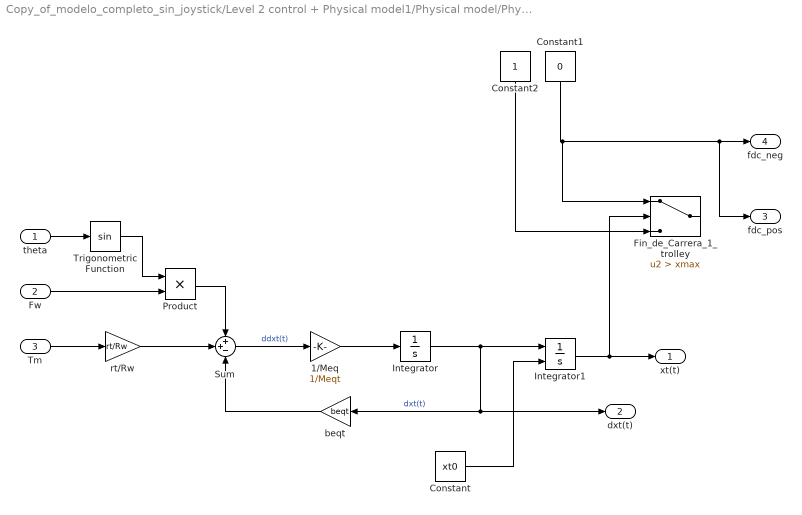
== system Copy_of_modelo_completo_sin_joystick/Level 2 control + Physical model1/Physical model/Physical Model/Trolley (carro) ==
  theta : Inport
  Fw : Inport  Port=2
  Tm : Inport  Port=3
  1/Meq : Gain  Gain=1/Meqt
  Constant : Constant  Value=xt0
  Constant1 : Constant  Value=0
  Constant2 : Constant
  Fin_de_Carrera_1_trolley : Switch  Criteria=u2 > Threshold  Threshold=xmax
  Integrator : Integrator
  Integrator1 : Integrator  InitialConditionSource=external
  Product : Product
  Sum : Sum  Inputs=++-
  Trigonometric Function : Trigonometry
  beqt : Gain  Gain=beqt
  rt/Rw : Gain  Gain=rt/Rw
  xt(t) : Outport
  dxt(t) : Outport  Port=2
  fdc_pos : Outport  Port=3
  fdc_neg : Outport  Port=4
  wires:
  theta/1 -> Trigonometric Function/1
  Trigonometric Function/1 -> Product/1
  Fw/1 -> Product/2
  Product/1 -> Sum/1
  Tm/1 -> rt/Rw/1
  rt/Rw/1 -> Sum/2
  Sum/1 -> 1/Meq/1  "ddxt(t)"
  1/Meq/1 -> Integrator/1
  Integrator/1 -> Integrator1/1, dxt(t)/1, beqt/1  "dxt(t)"
  beqt/1 -> Sum/3
  Constant/1 -> Integrator1/2
  Integrator1/1 -> Fin_de_Carrera_1_trolley/2, xt(t)/1
  Constant1/1 -> Fin_de_Carrera_1_trolley/1, fdc_pos/1, fdc_neg/1
  Constant2/1 -> Fin_de_Carrera_1_trolley/3

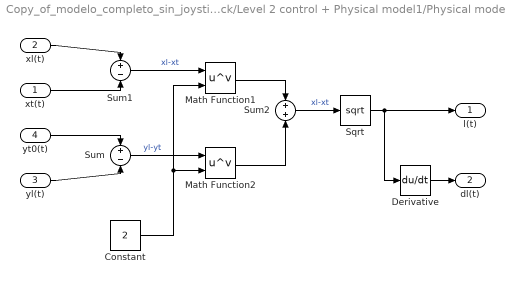
== system Copy_of_modelo_completo_sin_joystick/Level 2 control + Physical model1/Physical model/Physical Model/l (wire length) ==
  xt(t) : Inport
  xl(t) : Inport  Port=2
  yl(t) : Inport  Port=3
  yt0(t) : Inport  Port=4
  Constant : Constant  Value=2
  Derivative : Derivative
  Math Function1 : Math  Operator=pow  SignedPower=on  SaturateOnIntegerOverflow=on
  Math Function2 : Math  Operator=pow  SignedPower=on  SaturateOnIntegerOverflow=on
  Sqrt : Sqrt  SaturateOnIntegerOverflow=on
  Sum : Sum  Inputs=+-
  Sum1 : Sum  Inputs=+-
  Sum2 : Sum
  l(t) : Outport
  dl(t) : Outport  Port=2
  wires:
  yt0(t)/1 -> Sum/1
  yl(t)/1 -> Sum/2
  xl(t)/1 -> Sum1/1
  xt(t)/1 -> Sum1/2
  Sqrt/1 -> Derivative/1, l(t)/1
  Sum1/1 -> Math Function1/1  "xl-xt"
  Sum/1 -> Math Function2/1  "yl-yt"
  Math Function1/1 -> Sum2/1
  Math Function2/1 -> Sum2/2
  Sum2/1 -> Sqrt/1  "xl-xt"
  Derivative/1 -> dl(t)/1
  Constant/1 -> Math Function2/2, Math Function1/2
